simulink model "IP_Core_SS_Switch_and_PWM"  (R2021a)
settings: Solver=VariableStepAuto  StartTime=0.0  StopTime=0.001  RelTol=1e-3
values from neighbouring files (symbols this model uses):
  f_FPGA_clk = 100e6    (= 100000000)    [Init_IP_Core.m]
  T_FPGA_clk = 1/f_FPGA_clk    (= 1e-08)    [Init_IP_Core.m]
libraries: hdlsllib x4, simulink x2
(part 3 of 3)

== system IP_Core_SS_Switch_and_PWM/PWM_and_Switching_Signal_Control1/GenPWM/Triangle shift1/Subsystem3 ==
  triangle_in : Inport
  modified triangle_shift : Inport  Port=2
  direction up : Inport  Port=3
  Relational Operator6 : RelationalOperator  Operator=<=  OutDataTypeStr=boolean  RndMeth=Nearest
  Sum2 : Sum  Inputs=|-+
  Sum3 : Sum  Inputs=|+-
  Sum4 : Sum  Inputs=|++
  Switch3 : Switch  Criteria=u2 > Threshold
  sw : Switch  Criteria=u2 > Threshold
  shifted triangle_in signal : Outport
  wires:
  Sum4/1 -> sw/3
  modified triangle_shift/1 -> Sum4/1, Sum3/2, Sum2/2, Relational Operator6/2
  Switch3/1 -> sw/1
  Sum3/1 -> Switch3/3
  Sum2/1 -> Switch3/1
  sw/1 -> shifted triangle_in signal/1
  Relational Operator6/1 -> Switch3/2
  direction up/1 -> sw/2
  triangle_in/1 -> Relational Operator6/1, Sum3/1, Sum2/1, Sum4/2

== system IP_Core_SS_Switch_and_PWM/PWM_and_Switching_Signal_Control1/GenPWM/Triangle shift2/Subsystem ==
  note: AND block replaced with
      | switches for better performance
  Zero_input : Inport
  converted triangle_shift : Inport  Port=2
  modified triangle_shift : Inport  Port=3
  triangle_in : Inport  Port=4
  direction down : Inport  Port=5
  Relational Operator11 : RelationalOperator  Operator=<=  OutDataTypeStr=boolean  RndMeth=Nearest
  Sum8 : Sum  Inputs=|-+
  Unary Minus : UnaryMinus
  and2_1 : Switch  Criteria=u2 > Threshold
  and2_2 : Switch  Criteria=u2 > Threshold
  shifted triangle_in signal : Outport
  enable_out : Outport  Port=2
  wires:
  direction down/1 -> and2_2/2
  Zero_input/1 -> and2_1/3, and2_2/3
  Relational Operator11/1 -> and2_1/2
  and2_1/1 -> and2_2/1
  Sum8/1 -> shifted triangle_in signal/1
  Unary Minus/1 -> Sum8/2, Relational Operator11/2
  triangle_in/1 -> Sum8/1, Relational Operator11/1
  converted triangle_shift/1 -> and2_1/1
  and2_2/1 -> enable_out/1
  modified triangle_shift/1 -> Unary Minus/1

== system IP_Core_SS_Switch_and_PWM/PWM_and_Switching_Signal_Control1/GenPWM/Triangle shift2/Subsystem1 ==
  note: AND block replaced with
      | switches for better performance
  note: AND block replaced with
      | switches for better performance
  standardized peak of triangle : Inport
  triangle_in : Inport  Port=2
  converted triangle_shift : Inport  Port=3
  modified triangle_shift : Inport  Port=4
  Zero_input : Inport  Port=5
  direction up : Inport  Port=6
  Relational Operator2 : RelationalOperator  OutDataTypeStr=boolean  RndMeth=Nearest
  Sum11 : Sum  Inputs=++-  OutDataTypeStr=fixdt(1,21,17)
  Sum6 : Sum  Inputs=++|
  and1_1 : Switch  Criteria=u2 > Threshold
  and1_2 : Switch  Criteria=u2 > Threshold
  shifted triangle_in signal : Outport
  enable_out : Outport  Port=2
  wires:
  Sum11/1 -> shifted triangle_in signal/1
  Sum6/1 -> Relational Operator2/2, Sum11/2
  and1_1/1 -> and1_2/1
  Relational Operator2/1 -> and1_1/2
  Zero_input/1 -> and1_2/3, and1_1/3
  standardized peak of triangle/1 -> Sum6/2, Sum11/1
  and1_2/1 -> enable_out/1
  converted triangle_shift/1 -> and1_1/1
  direction up/1 -> and1_2/2
  triangle_in/1 -> Relational Operator2/1, Sum11/3
  modified triangle_shift/1 -> Sum6/1

== system IP_Core_SS_Switch_and_PWM/PWM_and_Switching_Signal_Control1/GenPWM/Triangle shift2/Subsystem2 ==
  triangle_in : Inport
  modified triangle_shift : Inport  Port=2
  standardized peak of triangle : Inport  Port=3
  Zero_input : Inport  Port=4
  direction down : Inport  Port=5
  Relational Operator9 : RelationalOperator  OutDataTypeStr=boolean  RndMeth=Nearest
  Sum1 : Sum  Inputs=|-+
  Sum5 : Sum  Inputs=++-  OutDataTypeStr=fixdt(1,21,17)
  and : Switch  Criteria=u2 > Threshold
  shifted triangle_in signal : Outport
  enable_out : Outport  Port=2
  wires:
  standardized peak of triangle/1 -> Sum1/2, Sum5/2
  Zero_input/1 -> and/3
  Sum1/1 -> Relational Operator9/2, Sum5/1
  Relational Operator9/1 -> and/1
  direction down/1 -> and/2
  and/1 -> enable_out/1
  triangle_in/1 -> Relational Operator9/1, Sum5/3
  Sum5/1 -> shifted triangle_in signal/1
  modified triangle_shift/1 -> Sum1/1

== system IP_Core_SS_Switch_and_PWM/PWM_and_Switching_Signal_Control1/GenPWM/Triangle shift2/Subsystem3 ==
  triangle_in : Inport
  modified triangle_shift : Inport  Port=2
  direction up : Inport  Port=3
  Relational Operator6 : RelationalOperator  Operator=<=  OutDataTypeStr=boolean  RndMeth=Nearest
  Sum2 : Sum  Inputs=|-+
  Sum3 : Sum  Inputs=|+-
  Sum4 : Sum  Inputs=|++
  Switch3 : Switch  Criteria=u2 > Threshold
  sw : Switch  Criteria=u2 > Threshold
  shifted triangle_in signal : Outport
  wires:
  Sum4/1 -> sw/3
  modified triangle_shift/1 -> Sum4/1, Sum3/2, Sum2/2, Relational Operator6/2
  Switch3/1 -> sw/1
  Sum3/1 -> Switch3/3
  Sum2/1 -> Switch3/1
  sw/1 -> shifted triangle_in signal/1
  Relational Operator6/1 -> Switch3/2
  direction up/1 -> sw/2
  triangle_in/1 -> Relational Operator6/1, Sum3/1, Sum2/1, Sum4/2
